simulink model "MBSE_Project_SeatBeltRemainder"  (R2020b)
settings: Solver=VariableStepAuto  StartTime=0.0  StopTime=inf  RelTol=1e-3
settings Model: Creator=99003747  LastModifiedBy=99003747

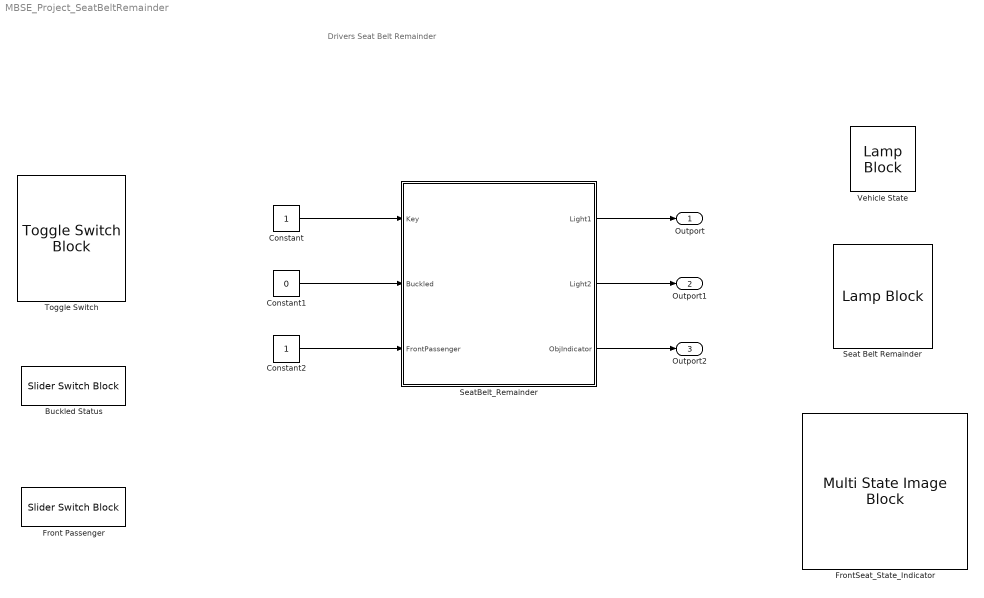
== system MBSE_Project_SeatBeltRemainder ==
  note: Drivers Seat Belt Remainder
  Buckled Status : SliderSwitchBlock
      settings: Values={{'Off', 'On'}, [0 1]}
  Constant : Constant
  Constant1 : Constant  Value=0
  Constant2 : Constant
  Front Passenger : SliderSwitchBlock
      settings: Values={{'Off', 'On'}, [0 1]}
  FrontSeat_State_Indicator : MultiStateImageBlock
  Seat Belt Remainder : LampBlock
  SeatBelt_Remainder : Stateflow chart  TreatAsAtomicUnit=on
  Toggle Switch : ToggleSwitchBlock
      settings: Values={{'Off', 'On'}, [0 1]}
  Vehicle State : LampBlock
  Outport : Outport
  Outport1 : Outport  Port=2
  Outport2 : Outport  Port=3
  wires:
  SeatBelt_Remainder/1(Light1) -> Outport/1
  SeatBelt_Remainder/2(Light2) -> Outport1/1
  Constant/1 -> SeatBelt_Remainder/1(Key)
  Constant1/1 -> SeatBelt_Remainder/2(Buckled)
  Constant2/1 -> SeatBelt_Remainder/3(FrontPassenger)
  SeatBelt_Remainder/3(ObjIndicator) -> Outport2/1

== stateflow chart MBSE_Project_SeatBeltRemainder/SeatBelt_Remainder ==
  state Indicator
    entry:
    ObjIndicator=1;
    state VehicleOn
      entry:
      Light1=1;
      Light2=1;
    state Chime
      entry:
      Light2=0;
    (default) -> VehicleOn
    Chime -> VehicleOn : [Light2==0]
    VehicleOn -> Chime : [Light2==1]
  state VehicleOff
    entry:
    Light1=0;
    Light2=0;
  state SeatBeltBuckled
    entry:
    Light2=0;
  state frontPassenger
    entry:
    ObjIndicator=0;
  (default) -> VehicleOff
  Indicator -> SeatBeltBuckled [order 1] : [Buckled==1]
  Indicator -> VehicleOff [order 3] : [Key==0]
  SeatBeltBuckled -> Indicator [order 1] : [Buckled==0]
  VehicleOff -> Indicator : [Key==1 ]
  SeatBeltBuckled -> VehicleOff [order 2] : [Key==0]
  frontPassenger -> SeatBeltBuckled [order 2] : [Buckled == 1]
  SeatBeltBuckled -> frontPassenger [order 3] : [Buckled == 0]
  frontPassenger -> Indicator [order 1] : [Key == 1 && FrontPassenger ==1 ]
  Indicator -> frontPassenger [order 2] : [ FrontPassenger ==0]
  frontPassenger -> VehicleOff [order 3] : [Key == 0]
  data: Light1 output; Light2 output; Key input =0; Buckled input; ObjIndicator output; FrontPassenger input
